simulink model "State_Space_Simulation_Sinusoid"  (R2019a)
settings: Solver=VariableStepAuto  StartTime=0.0  StopTime=40  RelTol=1e-3
values from neighbouring files (symbols this model uses):
  A = 1/5    (= 0.2)    [Pendulum_SS_Init.m]    (also in Pendulum_State_Space.m = [0, 1; -b, -a])
  a = 13.96    [Pendelum_TF2.mat]    (also in Pendulum_State_Space.m = 1)
  B = [0, c]'    [Pendulum_State_Space.m]
  C_lqi = [1 0]    [Pendulum_State_Space.m]
  G = [1, 0]'    [Pendulum_State_Space.m]
  K = K_joint(1:2)    [Pendulum_State_Space.m]
  omega = 1    [Pendulum_State_Space.m]
  phi = 0    [Pendulum_State_Space.m]
settings Model: Creator=QuarcUser  LastModifiedBy=QuarcUser

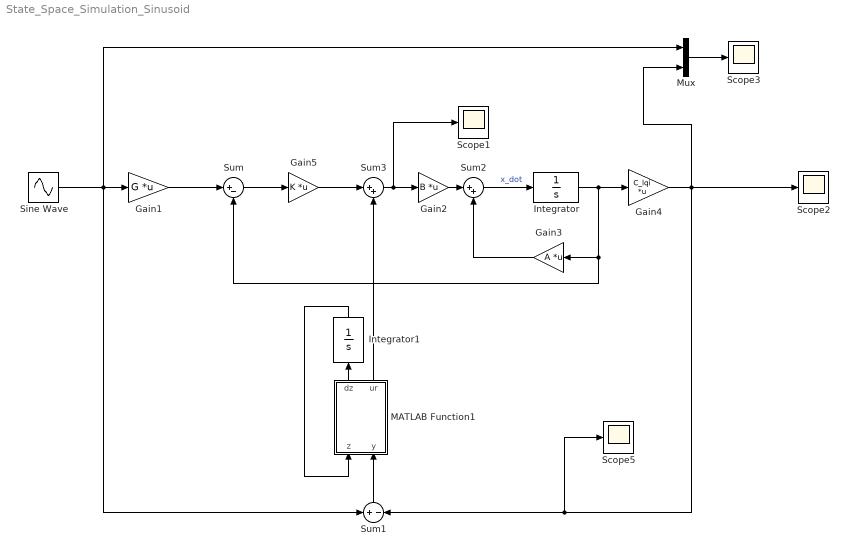
== system State_Space_Simulation_Sinusoid ==
  Gain1 : Gain  Gain=G  Multiplication=Matrix(K*u)
  Gain2 : Gain  Gain=B  Multiplication=Matrix(K*u)
  Gain3 : Gain  Gain=A  Multiplication=Matrix(K*u)
  Gain4 : Gain  Gain=C_lqi  Multiplication=Matrix(K*u)
  Gain5 : Gain  Gain=K  Multiplication=Matrix(K*u)
  Integrator : Integrator  InitialCondition=[0;0]
  Integrator1 : Integrator  InitialCondition=[0;0]
  MATLAB Function1 : MATLAB Function  TreatAsAtomicUnit=on
  Mux : Mux  Inputs=2
  Scope{1..3,5} (4 alike) : Scope
  Sine Wave : Sin  Amplitude=a  Frequency=omega  Phase=phi  SampleTime=0
  Sum : Sum  Inputs=|+-
  Sum1 : Sum  Inputs=+-
  Sum2 : Sum  Inputs=|++
  Sum3 : Sum  Inputs=|++
  wires:
  Sum/1 -> Gain5/1
  Gain2/1 -> Sum2/1
  Sum2/1 -> Integrator/1  "x_dot"
  Gain3/1 -> Sum2/2
  Sum1/1 -> MATLAB Function1/2(y)
  Integrator/1 -> Gain3/1, Sum/2, Gain4/1
  Gain1/1 -> Sum/1
  Sine Wave/1 -> Sum1/1, Mux/1, Gain1/1
  Sum3/1 -> Scope1/1, Gain2/1
  Gain5/1 -> Sum3/1
  Gain4/1 -> Scope5/1, Sum1/2, Mux/2, Scope2/1
  Integrator1/1 -> MATLAB Function1/1(z)
  MATLAB Function1/1(dz) -> Integrator1/1
  Mux/1 -> Scope3/1
  MATLAB Function1/2(ur) -> Sum3/2

== matlab function State_Space_Simulation_Sinusoid/MATLAB Function1 ==
  data: z input; y input; dz output; ur output; omega parameter
function [dz,ur] = fcn(z,y,omega)
    A = [0 omega; -omega 0];
    B = [1; 0];
    C = [1 0];
    D = 0;
    
    dz = A*z + B*y;
    ur = C*z + D*y;
end
